simulink model "MI_observador"  (R2015a)
settings: Solver=ode45  StartTime=0.0  StopTime=1.0  RelTol=1e-3
values from neighbouring files (symbols this model uses):
  FLrd_0 = FLr_dq_0    [MI_controle_W_I_T_inicio.m]    (also in MI_controle_W_I_inicio.m; MI_controle_W_I_startup_inicio.m; MI_controle_W_Inicio.m; MI_controle_W_T_I_startup_inicio.m)
  FLsd_0 = FluxLinkage_dq(1)    [MI_controle_W_I_T_inicio.m]    (also in MI_controle_W_I_inicio.m; MI_controle_W_I_startup_inicio.m; MI_controle_W_Inicio.m; MI_controle_W_T_I_startup_inicio.m)
  FLsq_0 = FluxLinkage_dq(2)    [MI_controle_W_I_T_inicio.m]    (also in MI_controle_W_I_inicio.m; MI_controle_W_I_startup_inicio.m; MI_controle_W_Inicio.m; MI_controle_W_T_I_startup_inicio.m)
  J = 0.025    [MI_controle_W_I_T_inicio.m]    (also in MI_controle_W_I_inicio.m; MI_controle_W_I_startup_inicio.m; MI_controle_W_Inicio.m; MI_controle_W_T_I_startup_inicio.m)
  Lm = Xm/Wsyn    (= 0.368708951496)    [MI_controle_W_I_T_inicio.m]    (also in MI_controle_W_I_inicio.m; MI_controle_W_I_startup_inicio.m; MI_controle_W_Inicio.m; MI_controle_W_T_I_startup_inicio.m)
  Lr = (Xlr + Xm)/Wsyn    (= 0.380831252995)    [MI_controle_W_I_T_inicio.m]    (also in MI_controle_W_I_inicio.m; MI_controle_W_I_startup_inicio.m; MI_controle_W_Inicio.m; MI_controle_W_T_I_startup_inicio.m)
  Minv = inv(M)    [MI_controle_W_I_T_inicio.m]    (also in MI_controle_W_I_inicio.m; MI_controle_W_I_startup_inicio.m; MI_controle_W_Inicio.m; MI_controle_W_T_I_startup_inicio.m)
  p = 4    [MI_controle_W_I_T_inicio.m]    (also in MI_controle_W_I_inicio.m; MI_controle_W_I_startup_inicio.m; MI_controle_W_Inicio.m; MI_controle_W_T_I_startup_inicio.m)
  Rs = 1.77    [MI_controle_W_I_T_inicio.m]    (also in MI_controle_W_I_inicio.m; MI_controle_W_I_startup_inicio.m; MI_controle_W_Inicio.m; MI_controle_W_T_I_startup_inicio.m)
  tau_r = Lr/Rr    (= 0.284202427608)    [MI_controle_W_I_T_inicio.m]    (also in MI_controle_W_I_inicio.m; MI_controle_W_I_startup_inicio.m; MI_controle_W_Inicio.m; MI_controle_W_T_I_startup_inicio.m)
  TL_0 = Tem_0    [MI_controle_W_I_T_inicio.m]    (also in MI_controle_W_I_inicio.m; MI_controle_W_I_startup_inicio.m = 0; MI_controle_W_Inicio.m; MI_controle_W_T_I_startup_inicio.m = 0)
  Va = VLLrms*sqrt(2/3)    [MI_controle_W_I_T_inicio.m]    (also in MI_controle_W_I_inicio.m; MI_controle_W_I_startup_inicio.m; MI_controle_W_Inicio.m; MI_controle_W_T_I_startup_inicio.m)
  Wmech_0 = (2/p)*(1-s)*Wsyn    (= 185.253435597)    [MI_controle_W_I_T_inicio.m]    (also in MI_controle_W_I_inicio.m; MI_controle_W_I_startup_inicio.m = 0; MI_controle_W_Inicio.m; MI_controle_W_T_I_startup_inicio.m = 0)
  Wsyn = 2*pi*f    (= 376.991118431)    [MI_controle_W_I_T_inicio.m]    (also in MI_controle_W_I_inicio.m; MI_controle_W_I_startup_inicio.m; MI_controle_W_Inicio.m; MI_controle_W_T_I_startup_inicio.m)
undefined symbols (not defined in the file or in its folder): thetar
settings Model: Creator=range  LastModifiedBy=range

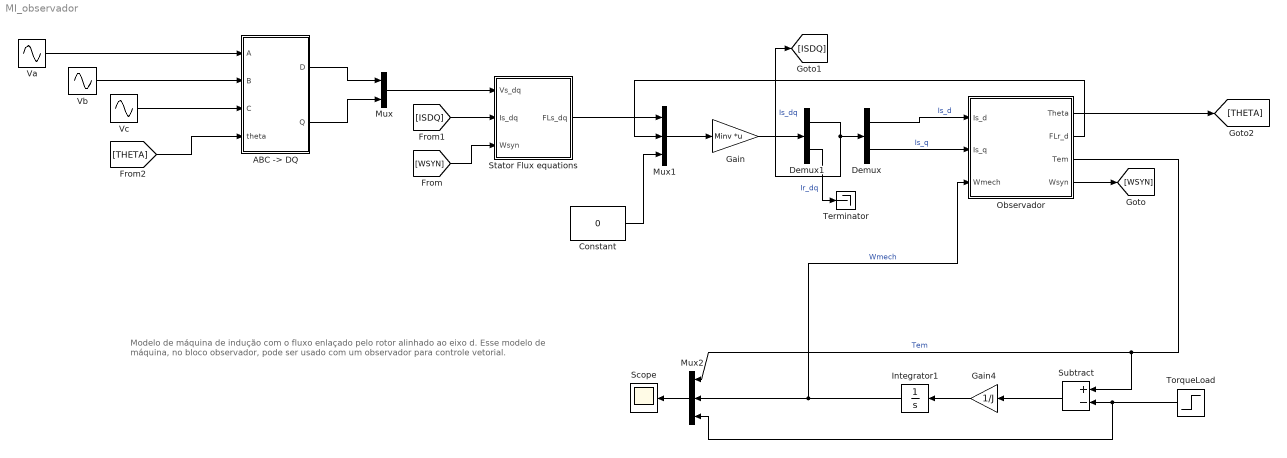
== system MI_observador ==
  note: Modelo de máquina de indução
      | com o fluxo enlaçado pelo rotor alinhado
      | ao eixo d.
      | Esse modelo de máquina, no bloco
      | observador, pode ser usado com um observador
      | para controle vetorial.
  "ABC -> DQ" : MATLAB Function  TreatAsAtomicUnit=on
  Constant : Constant  Value=0
  Demux : Demux  Outputs=2
  Demux1 : Demux  Outputs=2
  Gain : Gain  Gain=Minv  Multiplication=Matrix(K*u)
  Gain4 : Gain  Gain=1/J
  Integrator1 : Integrator  InitialCondition=Wmech_0
  Mux : Mux  Inputs=2
  Mux1 : Mux  Inputs=3
  Mux2 : Mux  Inputs=3
  Observador : Subsystem
  Scope : Scope
  Stator Flux equations : Subsystem
  Subtract : Sum  Inputs=+-
  Terminator : Terminator
  TorqueLoad : Step  Time=0.1  Before=TL_0  After=TL_0/2  SampleTime=0
  Va : Sin  Amplitude=Va  Frequency=Wsyn  Phase=pi/2  SampleTime=0
  Vb : Sin  Amplitude=Va  Frequency=Wsyn  Phase=pi/2-2*pi/3  SampleTime=0
  Vc : Sin  Amplitude=Va  Frequency=Wsyn  Phase=pi/2-4*pi/3  SampleTime=0
  wires:
  [THETA] -> "ABC -> DQ"/4(theta)
  Vc/1 -> "ABC -> DQ"/3(C)
  Vb/1 -> "ABC -> DQ"/2(B)
  Va/1 -> "ABC -> DQ"/1(A)
  "ABC -> DQ"/1(D) -> Mux/1
  "ABC -> DQ"/2(Q) -> Mux/2
  Mux/1 -> Stator Flux equations/1(Vs_dq)
  Mux1/1 -> Gain/1
  Stator Flux equations/1(FLs_dq) -> Mux1/1
  Gain4/1 -> Integrator1/1
  Subtract/1 -> Gain4/1
  TorqueLoad/1 -> Mux2/3, Subtract/2
  [WSYN] -> Stator Flux equations/3(Wsyn)
  Gain/1 -> Demux1/1
  Demux1/1 -> [ISDQ], Demux/1  "Is_dq"
  [ISDQ] -> Stator Flux equations/2(Is_dq)
  Constant/1 -> Mux1/3
  Demux1/2 -> Terminator/1  "Ir_dq"
  Observador/3(Tem) -> Subtract/1, Mux2/1  "Tem"
  Demux/1 -> Observador/1(Is_d)  "Is_d"
  Demux/2 -> Observador/2(Is_q)  "Is_q"
  Integrator1/1 -> Observador/3(Wmech), Mux2/2  "Wmech"
  Observador/1(Theta) -> [THETA]
  Observador/2(FLr_d) -> Mux1/2
  Observador/4(Wsyn) -> [WSYN]
  Mux2/1 -> Scope/1

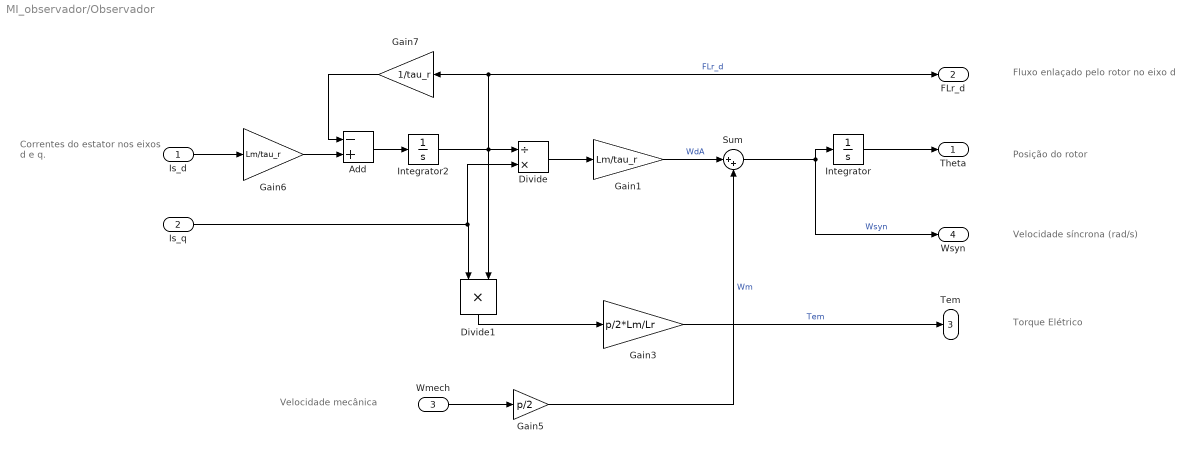
== system MI_observador/Observador ==
  note: Correntes do estator
      | nos eixos d e q.
  note: Velocidade mecânica
  note: Torque Elétrico
  note: Velocidade síncrona (rad/s)
  note: Posição do rotor
  note: Fluxo enlaçado pelo rotor no eixo d
  Is_d : Inport
  Is_q : Inport  Port=2
  Wmech : Inport  Port=3
  Add : Sum  Inputs=-+
  Divide : Product  Inputs=/*
  Divide1 : Product  Inputs=**
  Gain1 : Gain  Gain=Lm/tau_r
  Gain3 : Gain  Gain=p/2*Lm/Lr
  Gain5 : Gain  Gain=p/2
  Gain6 : Gain  Gain=Lm/tau_r
  Gain7 : Gain  Gain=1/tau_r
  Integrator : Integrator  InitialCondition=thetar
  Integrator2 : Integrator  InitialCondition=FLrd_0
  Sum : Sum  Inputs=|++
  Theta : Outport
  FLr_d : Outport  Port=2
  Tem : Outport  Port=3
  Wsyn : Outport  Port=4
  wires:
  Is_q/1 -> Divide/2, Divide1/1
  Integrator/1 -> Theta/1
  Sum/1 -> Wsyn/1, Integrator/1  "Wsyn"
  Add/1 -> Integrator2/1
  Gain1/1 -> Sum/1  "WdA"
  Is_d/1 -> Gain6/1
  Gain7/1 -> Add/1
  Gain6/1 -> Add/2
  Integrator2/1 -> Gain7/1, FLr_d/1, Divide1/2, Divide/1  "FLr_d"
  Divide1/1 -> Gain3/1
  Gain3/1 -> Tem/1  "Tem"
  Divide/1 -> Gain1/1
  Wmech/1 -> Gain5/1
  Gain5/1 -> Sum/2  "Wm"

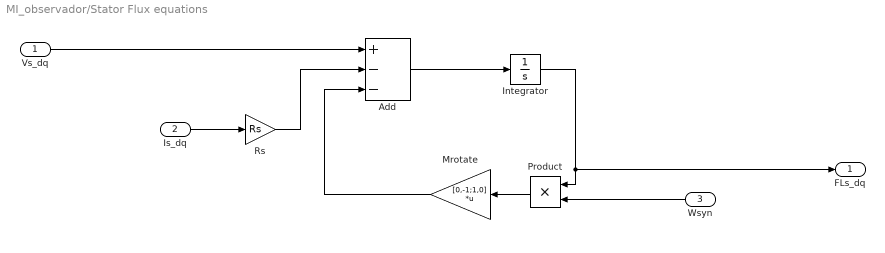
== system MI_observador/Stator Flux equations ==
  Vs_dq : Inport
  Is_dq : Inport  Port=2
  Wsyn : Inport  Port=3
  Add : Sum  Inputs=+--
  Integrator : Integrator  InitialCondition=[FLsd_0;FLsq_0]
  Mrotate : Gain  Gain=[0,-1;1,0]  Multiplication=Matrix(K*u)
  Product : Product
  Rs : Gain  Gain=Rs
  FLs_dq : Outport
  wires:
  Add/1 -> Integrator/1
  Is_dq/1 -> Rs/1
  Product/1 -> Mrotate/1
  Mrotate/1 -> Add/3
  Vs_dq/1 -> Add/1
  Rs/1 -> Add/2
  Integrator/1 -> FLs_dq/1, Product/1
  Wsyn/1 -> Product/2

== matlab function MI_observador/ABC -> DQ ==
  data: A input; D output; B input; C input; theta input; Q output
function [D,Q] = ABCtoDQ(A,B,C,theta)
%Transformação de grandezas trifásicas para os eixos D e Q.

DQ = sqrt(2/3)*[cos(theta), cos(theta-2*pi/3), cos(theta-4*pi/3);...
               -sin(theta),-sin(theta-2*pi/3),-sin(theta-4*pi/3)]*[A;B;C];
D = DQ(1);
Q = DQ(2);
